simulink model "q03_new"  (R2024a)
settings: Solver=FixedStepAuto  StartTime=0.0  StopTime=10  FixedStep=1/48  MaxStep=.1  RelTol=1e-6  EnableMultiTasking=on
settings Model: Creator=The MathWorks, Inc.  LastModifiedBy=amir
settings SolverCC: ConsecutiveZCsStepRelTol=1*128*eps  ZeroCrossControl=EnableAll  AlgebraicLoopSolver=TrustRegion  EnableFixedStepZeroCrossing=on
settings DataIOCC: SaveFormat=StructureWithTime  ReturnWorkspaceOutputs=off
settings OptimizationCC: ReuseModelBlockBuffer=off  ExpressionDepthLimit=2147483647  InitFltsAndDblsToZero=on  EfficientMapNaN2IntZero=off  LifeSpan=inf
settings DebuggingCC: UnderspecifiedInitializationDetection=Classic  MergeDetectMultiDrivingBlocksExec=none  SignalResolutionControl=TryResolveAllWithWarning  SolverPrmCheckMsg=warning  FcnCallInpInsideContextMsg=warning  UnconnectedInputMsg=warning  UnconnectedOutputMsg=warning  UnconnectedLineMsg=warning  StateNameClashWarn=warning  PregeneratedLibrarySubsystemCodeDiagnostic=none  SFUnexpectedBacktrackingDiag=warning  SFNoUnconditionalDefaultTransitionDiag=warning  SFExecutionAtInitializationDiag=none  ArithmeticOperatorsInVariantConditions=warning
settings HardwareCC: ProdBitPerPointer=32  ProdBitPerSizeT=32  ProdBitPerPtrDiffT=32  ProdLargestAtomicFloat=None  ProdIntDivRoundTo=Undefined  ProdEndianess=Unspecified  ProdWordSize=32  ProdHWDeviceType=32-bit Generic  TargetBitPerLong=64  TargetBitPerPointer=64  TargetBitPerSizeT=64  TargetBitPerPtrDiffT=64  TargetLongLongMode=on  TargetIntDivRoundTo=Zero  TargetEndianess=LittleEndian  TargetWordSize=64  TargetHWDeviceType=MATLAB Host
settings ModelReferenceCC: EnableRefExpFcnMdlSchedulingChecks=on  PropagateSignalLabelsOutOfModel=off
settings SFSimCC: SFSimEcho=off  SimUseLocalCustomCode=off  SimParseCustomCode=off  CustomCodeUndefinedFunction=UseInterfaceOnly
settings RTWCC: RTWUseLocalCustomCode=off  GPUComputeCapability=3.5  DLArmComputeVersion=19.05
settings CodeAppCC: StateflowObjectComments=on
settings GRTTargetCC: TargetLangStandard=C89/C90 (ANSI)  CombineOutputUpdateFcns=off  GRTInterface=on
settings ConfigComp: CovMetricSettings=dw  CovSaveCumulativeToWorkspaceVar=on  CovSaveSingleToWorkspaceVar=on  CovExternalEMLEnable=off  CovSFcnEnable=off

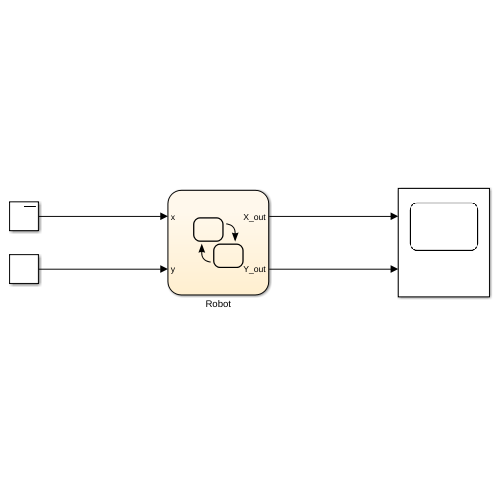
[thumbnail: Simulink's stored preview of the top-level diagram]
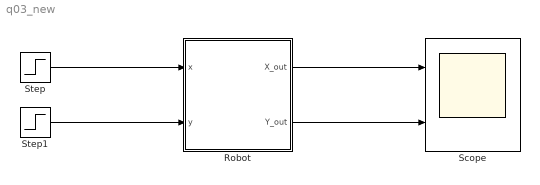
== system q03_new ==
  Robot : Stateflow chart  TreatAsAtomicUnit=on
  Scope : Scope  NumInputPorts=2
  Step : Step  After=4  SampleTime=0
  Step1 : Step  After=10  SampleTime=0
  wires:
  Robot/1(X_out) -> Scope/1
  Robot/2(Y_out) -> Scope/2
  Step/1 -> Robot/1(x)
  Step1/1 -> Robot/2(y)

== stateflow chart q03_new/Robot ==
  settings: updateMethod=CONTINUOUS  executeAtInitialization=1  initializeOutput=1
  state Down
    du:
    % derivatives
    X_dot = 0;
    Y_dot = -8;
    % outputs
    X_out = X;
    Y_out = Y;
  state Stopped
    du:
    % derivatives
    X_dot = 0;
    Y_dot = 0;
    % outputs
    X_out = X;
    Y_out = Y;
  state Up
    du:
    % derivatives
    X_dot = 0;
    Y_dot = 8;
    % outputs
    X_out = X;
    Y_out = Y;
  state Left
    du:
    % derivatives
    X_dot = -6;
    Y_dot = 0;
    % outputs
    X_out = X;
    Y_out = Y;
  state Straight
    du:
    % derivatives
    X_dot = 5*((x-X)/((X-x)^2+(Y-y)^2)^(0.5));
    Y_dot = 5*((y-Y)/((X-x)^2+(Y-y)^2)^(0.5));
    % outputs
    X_out = X;
    Y_out = Y;
  state Right
    du:
    % derivatives
    X_dot = 6;
    Y_dot = 0;
    % outputs
    X_out = X;
    Y_out = Y;
  (default) -> Stopped : {
      | X = 0;
      | Y = 0;
      | }
  Stopped -> Down [order 2] : [(abs(Y-y) >= 0.75 * abs(X-x)) && (y < Y) && abs(X-x)>=0.1 && abs(Y-y)>=0.1]
  Stopped -> Up [order 1] : [(abs(Y-y) >= 0.75 * abs(X-x)) && (y > Y) && abs(X-x)>=0.1 && abs(Y-y)>=0.1]
  Down -> Straight : [abs(Y-y) <= 0.75 * abs(X-x) && abs(X-x)>=0.1 && abs(Y-y)>=0.1]
  Stopped -> Left [order 4] : [(abs(Y-y) <= 0.75 * abs(X-x)) && (x > X)]
  Straight -> Stopped : [abs(X-x)<0.1 && abs(Y-y)<0.1]
  Stopped -> Right [order 3] : [(abs(Y-y) <= 0.75 * abs(X-x)) && (x > X)]
  Up -> Straight : [abs(Y-y) <= 0.75 * abs(X-x) && abs(X-x)>=0.1 && abs(Y-y)>=0.1]
  Left -> Straight : [abs(Y-y) >= 0.75 * abs(X-x)]
  Right -> Straight : [abs(Y-y) >= 0.75 * abs(X-x)]
  data: X_out output double size=1; X local double; Y local double; Y_out output double size=1; x input; y input
  data X settings: updateMethod=SF_CONTINUOUS_TIME_DATA
  data Y settings: updateMethod=SF_CONTINUOUS_TIME_DATA
